simulink model "c166_multitasking"  (Simulink 6.0)
settings: Solver=FixedStepDiscrete  SolverMode=MultiTasking  StartTime=0.0  StopTime=100  FixedStep=T_c166_multitasking  RelTol=1e-3
PreLoadFcn:
  | RTWConfigurationCB('preloadfcn', bdroot);T_c166_multitasking = 0.001;
InitFcn:
  | % START RTW CONFIGURATION CODE %
  | RTWConfigurationCB('rtw_target_initfcn',gcs);
  | % END RTW CONFIGURATION CODE %
undefined symbols (not defined in the file or in its folder): T_c166_multitasking
libraries: exprofilelib x8, c166drivers x3, canblocks x1
settings Model: Creator=The MathWorks Inc.  LastModifiedBy=batserve  ExtModeAutoUpdateStatusClock=off  BufferReuse=off  ProdHWDeviceType=Infineon C16x
settings DataIOCC: SignalLoggingName=sigsOut
settings OptimizationCC: InlineParams=on  InlineInvariantSignals=off  OptimizeBlockIOStorage=off  BufferReuse=off  EnforceIntegerDowncast=off  ExpressionFolding=off  FoldNonRolledExpr=off  LocalBlockOutputs=off  ZeroExternalMemoryAtStartup=off  ZeroInternalMemoryAtStartup=off  InitFltsAndDblsToZero=off  LifeSpan=1
settings DebuggingCC: CheckExecutionContextPreStartOutputMsg=on  CheckExecutionContextRuntimeOutputMsg=on  SolverPrmCheckMsg=none
settings HardwareCC: ProdBitPerInt=16  ProdEndianess=LittleEndian  ProdWordSize=16  ProdHWDeviceType=Infineon C16x  TargetHWDeviceType=32-bit Generic
settings RTWCC: SystemTargetFile=c166.tlc  TemplateMakefile=c166.tmf  ProcessScript=c166_make_rtw_hook
settings CodeAppCC: IgnoreCustomStorageClasses=off
settings STFCustomTargetCC: TargetFcnLib=ansi_tfl_tmw.mat  GenFloatMathFcnCalls=ANSI_C  GenerateSampleERTMain=on  IncludeMdlTerminateFcn=off  CombineOutputUpdateFcns=on  ERTCustomFileBanners=on  SupportAbsoluteTime=off  SupportNonFinite=off  SupportComplex=off  PurelyIntegerCode=on  SupportContinuousTime=off  SupportNonInlinedSFcns=off  SystemTargetFile=c166.tlc
settings ERTTargetCC: TargetFcnLib=ansi_tfl_tmw.mat  GenFloatMathFcnCalls=ANSI_C  GenerateSampleERTMain=on  IncludeMdlTerminateFcn=off  SupportAbsoluteTime=off  SupportNonFinite=off  SupportComplex=off  PurelyIntegerCode=on  RootIOFormat=Individual Arguments  ERTCustomFileTemplate=example_file_process.tlc  InitialValueSource=Model
settings CustomProperty: DataType=RTWOptions_EnumType__toolbox_rtw_targets_c166_c166_c166_BuildActionC166  Value=None
settings EnumStrPairs: String=Run_with_simulator

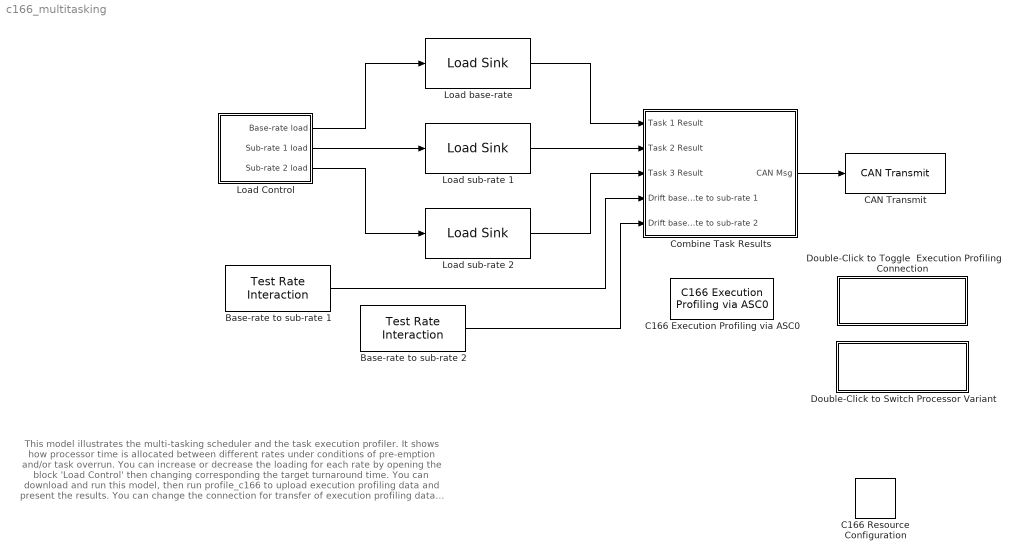
== system c166_multitasking ==
  note: This model illustrates the multi-tasking scheduler and the task execution profiler. It shows
      | how processor time is allocated between different rates under conditions of pre-emption
      | and/or task overrun.
      |
      | You can increase or decrease the loading for each rate by opening the block 'Load Control'
      | then changing corresponding the target turnaround time.
      |
      | You can download and run this model, then run profile_c166 to upload execution profiling
      | data  and present the results.  You can change the connection for transfer of execution
      | profiling data by double-clicking the convenience block.
  Base-rate to sub-rate 1 : exprofilelib/Test Rate Interaction  t=T_c166_multitasking
  Base-rate to sub-rate 2 : exprofilelib/Test Rate Interaction  t=T_c166_multitasking*4
  C166 Resource Configuration : c166drivers/C166 Resource Configuration  Tag=RTW CONFIGURATION BLOCK  Priority=-100000  oldParentName=c166_multitasking  oldBlockName=|  defaultConfigLibrary=c166drivers
      | c166_multitasking/C166
      | Resource
      | Configuration
  C166 Execution Profiling via ASC0 : c166drivers/Execution Profiling/C166 Execution Profiling via ASC0  t=T_c166_multitasking*4  execCopyFcn=on
  CAN Transmit : c166drivers/CAN Interface/CAN Transmit  module=A  tx_mode=Queued transmission with shared buffer  fifo_queue_length=8  buffer_select_mode=Automatic  bufferids=0  t=-1  irq_level=0
  Combine Task Results : Subsystem  PropExecContextAcrossSSBoundary=on
  Double-Click to Switch Processor Variant : Subsystem  PropExecContextAcrossSSBoundary=on
      settings: OpenFcn=c166switchconfig(gcs)
      mask Display: disp('Switch Target\nProcessor Variant');
  Double-Click to Toggle  Execution Profiling Connection : Subsystem  TreatAsAtomicUnit=on  PropExecContextAcrossSSBoundary=on
      settings: OpenFcn=toggle_exprofiling_c166(gcs);
      mask Display: disp('Switch Execution\nProfiling Connection')
  Load Control : Subsystem  PropExecContextAcrossSSBoundary=on
  Load base-rate : exprofilelib/Load Sink  mode=int16  t=T_c166_multitasking
  Load sub-rate 1 : exprofilelib/Load Sink  mode=int16  t=T_c166_multitasking*4
  Load sub-rate 2 : exprofilelib/Load Sink  mode=int16  t=T_c166_multitasking*16
  wires:
  Load Control/1(Base-rate load) -> Load base-rate/1
  Load base-rate/1 -> Combine Task Results/1(Task 1 Result)
  Load Control/2(Sub-rate 1 load) -> Load sub-rate 1/1
  Load Control/3(Sub-rate 2 load) -> Load sub-rate 2/1
  Load sub-rate 1/1 -> Combine Task Results/2(Task 2 Result)
  Load sub-rate 2/1 -> Combine Task Results/3(Task 3 Result)
  Combine Task Results/1(CAN Msg) -> CAN Transmit/1
  Base-rate to sub-rate 1/1 -> Combine Task Results/4(Drift base-rate to sub-rate 1)
  Base-rate to sub-rate 2/1 -> Combine Task Results/5(Drift base-rate to sub-rate 2)

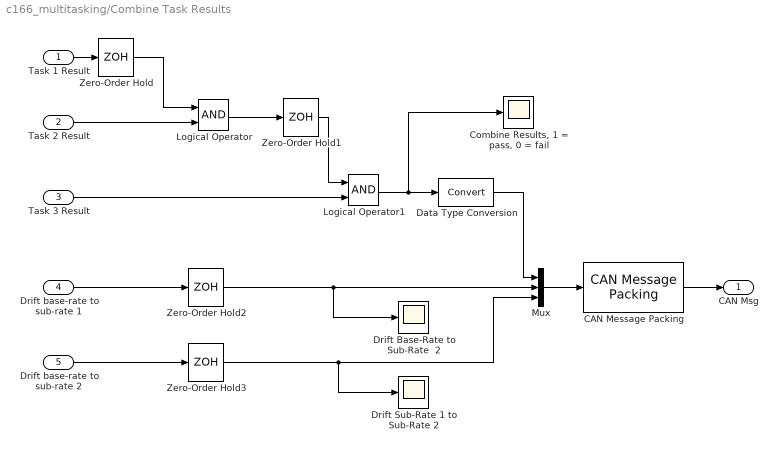
== system c166_multitasking/Combine Task Results ==
  Task 1 Result : Inport  Port=1  LatchInput=off
  Task 2 Result : Inport  Port=2  LatchInput=off
  Task 3 Result : Inport  Port=3  LatchInput=off
  Drift base-rate to sub-rate 1 : Inport  Port=4  LatchInput=off
  Drift base-rate to sub-rate 2 : Inport  Port=5  LatchInput=off
  CAN Message Packing : canblocks/CAN Message Packing  id=hex2dec('1')  message_type=Extended (29-bit identifier)  endian=Big Endian (Motorola)
  "Combine Results, 1 = pass, 0 = fail" : Scope
      settings: TimeRange=0.1  YMin=0.95  YMax=1.05  SaveName=ScopeData12
  Data Type Conversion : DataTypeConversion  OutDataTypeMode=uint8  RndMeth=Zero
  Drift Base-Rate to Sub-Rate  2 : Scope
      settings: TimeRange=20  YMin=-1  YMax=1
  Drift Sub-Rate 1 to Sub-Rate 2 : Scope
      settings: TimeRange=20  YMin=-1  YMax=1
  Logical Operator : Logic  AllPortsSameDT=off
  Logical Operator1 : Logic  AllPortsSameDT=off
  Mux : Mux  Inputs=3
  Zero-Order Hold : ZeroOrderHold  SampleTime=T_c166_multitasking*4
  Zero-Order Hold1 : ZeroOrderHold  SampleTime=T_c166_multitasking*16
  Zero-Order Hold2 : ZeroOrderHold  SampleTime=T_c166_multitasking*16
  Zero-Order Hold3 : ZeroOrderHold  SampleTime=T_c166_multitasking*16
  CAN Msg : Outport
  wires:
  Zero-Order Hold/1 -> Logical Operator/1
  Logical Operator/1 -> Zero-Order Hold1/1
  Logical Operator1/1 -> "Combine Results, 1 = pass, 0 = fail"/1, Data Type Conversion/1
  Zero-Order Hold1/1 -> Logical Operator1/1
  CAN Message Packing/1 -> CAN Msg/1
  Task 1 Result/1 -> Zero-Order Hold/1
  Task 2 Result/1 -> Logical Operator/2
  Task 3 Result/1 -> Logical Operator1/2
  Mux/1 -> CAN Message Packing/1
  Data Type Conversion/1 -> Mux/1
  Drift base-rate to sub-rate 1/1 -> Zero-Order Hold2/1
  Drift base-rate to sub-rate 2/1 -> Zero-Order Hold3/1
  Zero-Order Hold2/1 -> Drift Base-Rate to Sub-Rate  2/1, Mux/2
  Zero-Order Hold3/1 -> Mux/3, Drift Sub-Rate 1 to Sub-Rate 2/1

== system c166_multitasking/Double-Click to Switch Processor Variant ==

== system c166_multitasking/Double-Click to Toggle  Execution Profiling Connection ==

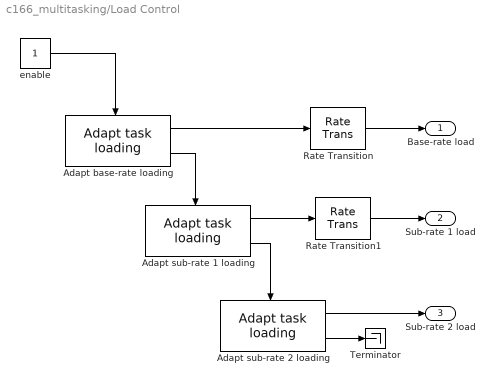
== system c166_multitasking/Load Control ==
  Adapt base-rate loading : exprofilelib/Adapt task loading  rateNum=0  target=uint16(2500)  adapt=4  t=T_c166_multitasking*16
  Adapt sub-rate 1 loading : exprofilelib/Adapt task loading  rateNum=1  target=uint16(10000)  adapt=16  t=T_c166_multitasking*16
  Adapt sub-rate 2 loading : exprofilelib/Adapt task loading  rateNum=2  target=uint16(40000)  adapt=64  t=T_c166_multitasking*16
  Rate Transition : RateTransition
  Rate Transition1 : RateTransition
  Terminator : Terminator
  enable : Constant  OutDataTypeMode=boolean
  Base-rate load : Outport
  Sub-rate 1 load : Outport  Port=2
  Sub-rate 2 load : Outport  Port=3
  wires:
  Rate Transition/1 -> Base-rate load/1
  Adapt base-rate loading/1 -> Rate Transition/1
  enable/1 -> Adapt base-rate loading/Enable
  Adapt base-rate loading/2 -> Adapt sub-rate 1 loading/Enable
  Rate Transition1/1 -> Sub-rate 1 load/1
  Adapt sub-rate 1 loading/1 -> Rate Transition1/1
  Adapt sub-rate 1 loading/2 -> Adapt sub-rate 2 loading/Enable
  Adapt sub-rate 2 loading/1 -> Sub-rate 2 load/1
  Adapt sub-rate 2 loading/2 -> Terminator/1
